simulink model "SD_Linear_n9960210"  (R2021a)
settings: Solver=VariableStepAuto  StartTime=0.0  StopTime=10.0  RelTol=1e-3
values from neighbouring files (symbols this model uses):
  A = [0 1 0 ... (first row only)    [main_n9960210_plotall.m]
  B = [0 ... (first row only)    [main_n9960210_plotall.m]
  C = [1 0 0]    [main_n9960210_plotall.m]
  D = 0    [main_n9960210_plotall.m]
  u_bar = 1    [main_n9960210_plotall.m]
  x_bar = [2*u_bar-1 ... (first row only)    [main_n9960210_plotall.m]
undefined symbols (not defined in the file or in its folder): Kd, x0_tilde
settings Model: Creator=isaac  LastModifiedBy=isaac

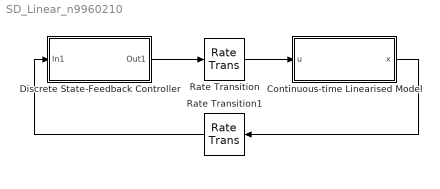
== system SD_Linear_n9960210 ==
  Continuous-time Linearised Model : Subsystem
  Discrete State-Feedback Controller : Subsystem
  Rate Transition : RateTransition  InitialCondition=-Kd*x0_tilde
  Rate Transition1 : RateTransition  InitialCondition=x0_tilde  OutPortSampleTime=Ts
  wires:
  Discrete State-Feedback Controller/1(Out1) -> Rate Transition/1
  Rate Transition/1 -> Continuous-time Linearised Model/1(u)
  Continuous-time Linearised Model/1(x) -> Rate Transition1/1
  Rate Transition1/1 -> Discrete State-Feedback Controller/1(In1)

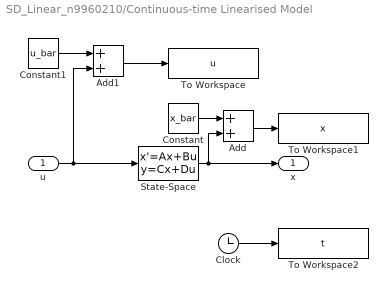
== system SD_Linear_n9960210/Continuous-time Linearised Model ==
  u : Inport
  Add : Sum
  Add1 : Sum
  Clock : Clock
  Constant : Constant  Value=x_bar
  Constant1 : Constant  Value=u_bar
  State-Space : StateSpace  A=A  B=B  C=C  D=D  InitialCondition=x0_tilde
  To Workspace : ToWorkspace  VariableName=u  SampleTime=-1
  To Workspace1 : ToWorkspace  VariableName=x  SampleTime=-1
  To Workspace2 : ToWorkspace  VariableName=t  SampleTime=-1
  x : Outport
  wires:
  u/1 -> Add1/2, State-Space/1
  Clock/1 -> To Workspace2/1
  State-Space/1 -> Add/2, x/1
  Constant/1 -> Add/1
  Add/1 -> To Workspace1/1
  Constant1/1 -> Add1/1
  Add1/1 -> To Workspace/1

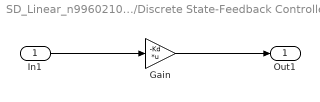
== system SD_Linear_n9960210/Discrete State-Feedback Controller ==
  In1 : Inport
  Gain : Gain  Gain=-Kd  Multiplication=Matrix(K*u)
  Out1 : Outport
  wires:
  In1/1 -> Gain/1
  Gain/1 -> Out1/1
